simulink model "massbalancer3"  (R2024a)
settings: Solver=ode45  StartTime=0.0  StopTime=300  MaxStep=0.5  RelTol=1e-3
libraries: matrix_library x29, sharedutil x3, sharedtransform x2, dspinverses x1, aerolibutil x1
(part 2 of 3)

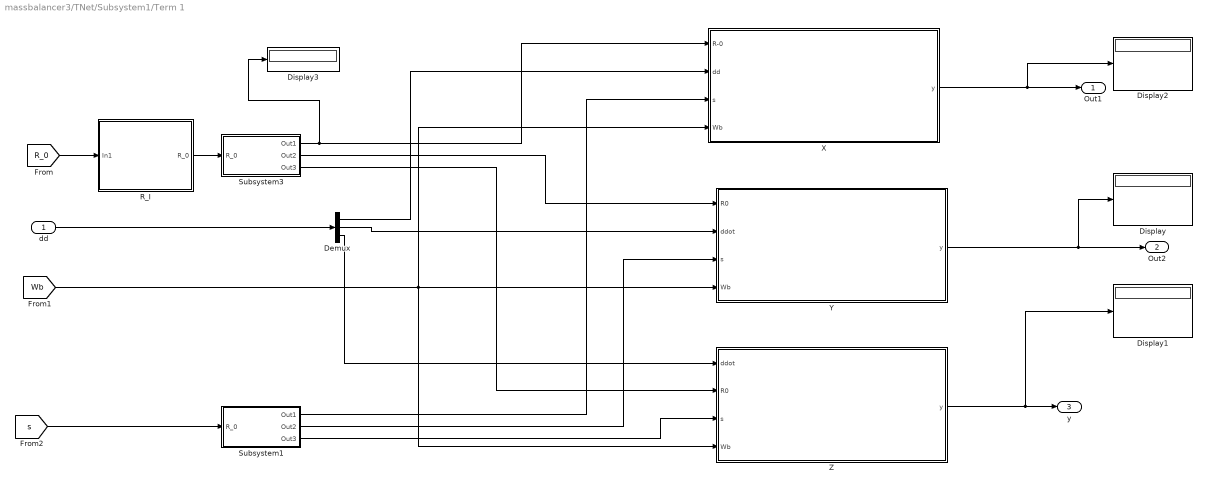
== system massbalancer3/TNet/Subsystem1/Term 1 ==
  dd : Inport
  Demux : Demux  Outputs=3
  Display{,1..3} (4 alike) : Display
  R_I : Subsystem
  Subsystem1 : Subsystem
  Subsystem3 : Subsystem
  X : Subsystem
  Y : Subsystem
  Z : Subsystem
  Out1 : Outport
  Out2 : Outport  Port=2
  y : Outport  Port=3
  wires:
  [R_0] -> R_I/1(In1)
  [s] -> Subsystem1/1(R_0)
  Demux/1 -> X/2(dd)
  R_I/1(R_0) -> Subsystem3/1(R_0)
  Subsystem3/1(Out1) -> X/1(R-0), Display3/1
  Subsystem1/2(Out2) -> Y/3(s)
  Subsystem1/1(Out1) -> X/3(s)
  Subsystem1/3(Out3) -> Z/3(s)
  Subsystem3/3(Out3) -> Z/2(R0)
  dd/1 -> Demux/1
  Subsystem3/2(Out2) -> Y/1(R0)
  Demux/3 -> Z/1(ddot)
  [Wb] -> X/4(Wb), Z/4(Wb), Y/4(Wb)
  Y/1(y) -> Display/1, Out2/1
  X/1(y) -> Display2/1, Out1/1
  Demux/2 -> Y/2(ddot)
  Z/1(y) -> Display1/1, y/1

== system massbalancer3/TNet/Subsystem1/Term2 ==
  dd : Inport
  Demux : Demux  Outputs=3
  Display : Display
  R_I : Subsystem
  Subsystem1 : Subsystem
  Subsystem3 : Subsystem
  X : Subsystem
  Y : Subsystem
  Z : Subsystem
  Output : Outport
  Output1 : Outport  Port=2
  Output2 : Outport  Port=3
  wires:
  Subsystem1/1(Out1) -> X/3(s)
  Demux/1 -> X/2(Ddot)
  dd/1 -> Demux/1
  Subsystem3/1(Out1) -> X/1(R-0)
  Demux/2 -> Y/2(ddot)
  Subsystem3/3(Out3) -> Z/2(R0)
  Subsystem3/2(Out2) -> Y/1(R0)
  [Wb] -> Z/4(Wb), X/4(Wb), Y/4(Wb)
  Demux/3 -> Z/1(ddot)
  [s] -> Subsystem1/1(R_0)
  Subsystem1/2(Out2) -> Y/3(s)
  [R_0] -> R_I/1(In1)
  Subsystem1/3(Out3) -> Z/3(s)
  X/1(Output) -> Output/1
  Y/1(Output) -> Display/1, Output1/1
  Z/1(Output1) -> Output2/1
  R_I/1(R_0) -> Subsystem3/1(R_0)

== system massbalancer3/TNet/Subsystem1/Term3 ==
  Input : Inport
  Demux : Demux  Outputs=3
  Display{,1..3} (4 alike) : Display
  Subsystem1 : Subsystem
  Subsystem3 : Subsystem
  X : Subsystem
  Y : Subsystem
  Z : Subsystem
  Output : Outport
  Output1 : Outport  Port=2
  Output2 : Outport  Port=3
  wires:
  Subsystem3/1(Out1) -> X/3(r)
  Subsystem3/2(Out2) -> Y/3(r)
  Subsystem3/3(Out3) -> Z/1(r)
  Demux/1 -> X/1(ddoubledot)
  Demux/2 -> Y/1(ddoubledot)
  Demux/3 -> Z/3(ddoubledot)
  [s] -> Subsystem1/1(R_0)
  Subsystem1/1(Out1) -> X/2(s)
  Subsystem1/2(Out2) -> Y/2(s)
  Subsystem1/3(Out3) -> Z/2(s)
  X/1(y) -> Display2/1, Output/1
  Y/1(y) -> Display/1, Output1/1
  Z/1(y) -> Display1/1, Output2/1
  [R_0] -> Subsystem3/1(R_0), Display3/1
  Input/1 -> Demux/1

== system massbalancer3/TNet/TBalances/R_I ==
  In1 : Inport
  Add : Sum
  Matrix Concatenate1 : Concatenate  NumInputs=3  Mode=Multidimensional array  ConcatenateDimension=2
  Product : Product
  Product1 : Product
  Product2 : Product
  Selector : Selector  InputPortWidth=3  IndexOptions=Index vector (dialog)  Indices=[1]  OutputSizes=1
  Selector1 : Selector  InputPortWidth=3  IndexOptions=Index vector (dialog)  Indices=[2]  OutputSizes=1
  Selector2 : Selector  InputPortWidth=3  IndexOptions=Index vector (dialog)  Indices=[3]  OutputSizes=1
  Subsystem3 : Subsystem
  Subsystem4 : Subsystem
  Sum1 : Sum  Inputs=|++
  Sum2 : Sum  Inputs=|++
  R_0 : Outport
  wires:
  Subsystem4/1(Out1) -> Add/1
  Product1/1 -> Sum1/1
  Selector1/1 -> Product1/1
  Selector/1 -> Product/1
  Subsystem3/2(Out2) -> Product1/2
  Selector2/1 -> Product2/1
  Subsystem4/2(Out2) -> Sum1/2
  In1/1 -> Selector/1, Selector1/1, Selector2/1
  Subsystem4/3(Out3) -> Sum2/2
  Product/1 -> Add/2
  Subsystem3/1(Out1) -> Product/2
  [S] -> Subsystem3/1(In1)
  Subsystem3/3(Out3) -> Product2/2
  Product2/1 -> Sum2/1
  [R_0] -> Subsystem4/1(In1)
  Add/1 -> Matrix Concatenate1/1
  Sum1/1 -> Matrix Concatenate1/2
  Sum2/1 -> Matrix Concatenate1/3
  Matrix Concatenate1/1 -> R_0/1

== system massbalancer3/TNet/TBalances/Term1 ==
  dd : Inport
  S : Inport  Port=2
  R_0 : Inport  Port=3
  Wb : Inport  Port=4
  Demux : Demux  Outputs=3
  Subsystem1 : Subsystem
  Subsystem3 : Subsystem
  X : Subsystem
  Y : Subsystem
  Z : Subsystem
  Output : Outport
  Output1 : Outport  Port=2
  Output2 : Outport  Port=3
  wires:
  R_0/1 -> Subsystem3/1(R_0)
  Subsystem3/1(Out1) -> X/1(R-0)
  Subsystem3/2(Out2) -> Y/1(R0)
  Subsystem3/3(Out3) -> Z/2(R0)
  dd/1 -> Demux/1
  Demux/1 -> X/2(dd)
  Demux/2 -> Y/2(ddot)
  Wb/1 -> Z/4(Wb), X/4(Wb), Y/4(Wb)
  Demux/3 -> Z/1(ddot)
  S/1 -> Subsystem1/1(R_0)
  Subsystem1/1(Out1) -> X/3(s)
  Subsystem1/2(Out2) -> Y/3(s)
  Subsystem1/3(Out3) -> Z/3(s)
  X/1(y) -> Output/1
  Y/1(y) -> Output1/1
  Z/1(y) -> Output2/1

== system massbalancer3/TNet/TBalances/Term2 ==
  ddot : Inport
  r0 : Inport  Port=2
  s : Inport  Port=3
  wb : Inport  Port=4
  Demux : Demux  Outputs=3
  Display : Display
  Display2 : Display
  Subsystem1 : Subsystem
  Subsystem3 : Subsystem
  X : Subsystem
  Y : Subsystem
  Z : Subsystem
  Output : Outport
  Output1 : Outport  Port=2
  Output2 : Outport  Port=3
  wires:
  Subsystem1/1(Out1) -> X/3(s)
  Demux/1 -> X/2(Ddot)
  ddot/1 -> Demux/1
  Subsystem3/1(Out1) -> X/1(R-0)
  Demux/2 -> Y/2(ddot)
  Subsystem3/3(Out3) -> Z/2(R0)
  Subsystem3/2(Out2) -> Y/1(R0)
  wb/1 -> Z/4(Wb), X/4(Wb), Y/4(Wb)
  Demux/3 -> Z/1(ddot)
  s/1 -> Subsystem1/1(R_0)
  Subsystem1/2(Out2) -> Y/3(s)
  r0/1 -> Subsystem3/1(R_0)
  Subsystem1/3(Out3) -> Z/3(s)
  X/1(Output) -> Display2/1, Output/1
  Y/1(Output) -> Output1/1
  Z/1(Output1) -> Display/1, Output2/1

== system massbalancer3/TNet/TBalances/Term3 ==
  r : Inport
  ddoubledot : Inport  Port=2
  s : Inport  Port=3
  Demux : Demux  Outputs=3
  Display : Display
  Display1 : Display
  Display2 : Display
  Subsystem1 : Subsystem
  Subsystem3 : Subsystem
  X : Subsystem
  Y : Subsystem
  Z : Subsystem
  Output : Outport
  Output1 : Outport  Port=2
  Output2 : Outport  Port=3
  wires:
  r/1 -> Subsystem3/1(R_0)
  ddoubledot/1 -> Demux/1
  Subsystem3/1(Out1) -> X/3(r)
  Subsystem3/2(Out2) -> Y/3(r)
  Subsystem3/3(Out3) -> Z/1(r)
  Demux/1 -> X/1(ddoubledot)
  Demux/2 -> Y/1(ddoubledot)
  Demux/3 -> Z/3(ddoubledot)
  s/1 -> Subsystem1/1(R_0)
  Subsystem1/1(Out1) -> X/2(s)
  Subsystem1/2(Out2) -> Y/2(s)
  Subsystem1/3(Out3) -> Z/2(s)
  X/1(y) -> Display2/1, Output/1
  Y/1(y) -> Display/1, Output1/1
  Z/1(y) -> Display1/1, Output2/1

== system massbalancer3/TNet/Tbalances Init T Gravity /Fgravity ==
  Matrix Multiply : Product  Multiplication=Matrix(*)
  Q(q) rotational form of quaternio : Subsystem
  Out1 : Outport
  wires:
  Q(q) rotational form of quaternio/1(Out1) -> Matrix Multiply/1
  [G] -> Matrix Multiply/2
  [q] -> Q(q) rotational form of quaternio/1(Q_input)
  Matrix Multiply/1 -> Out1/1

== system massbalancer3/TNet/Tbalances Init T Gravity /Subsystem ==
  Subsystem2 : Subsystem
  Output : Outport
  wires:
  [M_r] -> Subsystem2/1(In1)
  Subsystem2/1(Output) -> Output/1

== system massbalancer3/Wdot b/I_r/Subsystem ==
  In1 : Inport
  Constant : Constant  Value=0  VectorParams1D=off
  Constant1 : Constant  Value=0  VectorParams1D=off
  Constant2 : Constant  Value=0  VectorParams1D=off
  Demux : Demux  Outputs=3
  Gain : Gain  Gain=-1
  Gain1 : Gain  Gain=-1
  Gain2 : Gain  Gain=-1
  Matrix Concatenate : Concatenate  NumInputs=3  Mode=Multidimensional array  ConcatenateDimension=2
  Mux : Mux  Inputs=3
  Mux1 : Mux  Inputs=3
  Mux2 : Mux  Inputs=3
  Out1 : Outport
  wires:
  Constant/1 -> Mux/1
  Gain2/1 -> Mux2/1
  Gain1/1 -> Mux1/3
  Mux/1 -> Matrix Concatenate/1
  Demux/2 -> Mux/3, Gain2/1
  In1/1 -> Demux/1
  Gain/1 -> Mux/2
  Demux/3 -> Mux1/1, Gain/1
  Mux1/1 -> Matrix Concatenate/2
  Mux2/1 -> Matrix Concatenate/3
  Demux/1 -> Mux2/2, Gain1/1
  Constant1/1 -> Mux1/2
  Constant2/1 -> Mux2/3
  Matrix Concatenate/1 -> Out1/1

== system massbalancer3/Wdot b/I_r/Subsystem1 ==
  In1 : Inport
  Constant : Constant  Value=0  VectorParams1D=off
  Constant1 : Constant  Value=0  VectorParams1D=off
  Constant2 : Constant  Value=0  VectorParams1D=off
  Demux : Demux  Outputs=3
  Gain : Gain  Gain=-1
  Gain1 : Gain  Gain=-1
  Gain2 : Gain  Gain=-1
  Matrix Concatenate : Concatenate  NumInputs=3  Mode=Multidimensional array  ConcatenateDimension=2
  Mux : Mux  Inputs=3
  Mux1 : Mux  Inputs=3
  Mux2 : Mux  Inputs=3
  Out1 : Outport
  wires:
  Matrix Concatenate/1 -> Out1/1
  Constant2/1 -> Mux2/3
  Constant1/1 -> Mux1/2
  Demux/1 -> Gain1/1, Mux2/2
  Mux2/1 -> Matrix Concatenate/3
  Mux1/1 -> Matrix Concatenate/2
  Demux/3 -> Gain/1, Mux1/1
  Gain/1 -> Mux/2
  In1/1 -> Demux/1
  Demux/2 -> Gain2/1, Mux/3
  Mux/1 -> Matrix Concatenate/1
  Gain1/1 -> Mux1/3
  Gain2/1 -> Mux2/1
  Constant/1 -> Mux/1

== system massbalancer3/Wdot b/I_r/Subsystem2 ==
  In1 : Inport
  Constant : Constant  Value=0  VectorParams1D=off
  Constant1 : Constant  Value=0  VectorParams1D=off
  Constant2 : Constant  Value=0  VectorParams1D=off
  Demux : Demux  Outputs=3
  Gain : Gain  Gain=-1
  Gain1 : Gain  Gain=-1
  Gain2 : Gain  Gain=-1
  Matrix Concatenate : Concatenate  NumInputs=3  Mode=Multidimensional array  ConcatenateDimension=2
  Mux : Mux  Inputs=3
  Mux1 : Mux  Inputs=3
  Mux2 : Mux  Inputs=3
  Out1 : Outport
  wires:
  Constant/1 -> Mux/1
  Gain2/1 -> Mux2/1
  Gain1/1 -> Mux1/3
  Mux/1 -> Matrix Concatenate/1
  Demux/2 -> Mux/3, Gain2/1
  In1/1 -> Demux/1
  Gain/1 -> Mux/2
  Demux/3 -> Mux1/1, Gain/1
  Mux1/1 -> Matrix Concatenate/2
  Mux2/1 -> Matrix Concatenate/3
  Demux/1 -> Mux2/2, Gain1/1
  Constant1/1 -> Mux1/2
  Constant2/1 -> Mux2/3
  Matrix Concatenate/1 -> Out1/1

== system massbalancer3/Wdot b/I_r/Subsystem3 ==
  In1 : Inport
  Reshape : Reshape  OutputDimensionality=Column vector (2-D)  OutputDimensions=[1,3]
  Selector : Selector  InputPortWidth=9  IndexOptions=Index vector (dialog)  Indices=[1]  OutputSizes=1
  Selector1 : Selector  InputPortWidth=9  IndexOptions=Index vector (dialog)  Indices=[2]  OutputSizes=1
  Selector2 : Selector  InputPortWidth=9  IndexOptions=Index vector (dialog)  Indices=[3]  OutputSizes=1
  Selector3 : Selector  InputPortWidth=9  IndexOptions=Index vector (dialog)  Indices=[4]  OutputSizes=1
  Selector4 : Selector  InputPortWidth=9  IndexOptions=Index vector (dialog)  Indices=[5]  OutputSizes=1
  Selector5 : Selector  InputPortWidth=9  IndexOptions=Index vector (dialog)  Indices=[6]  OutputSizes=1
  Selector6 : Selector  InputPortWidth=9  IndexOptions=Index vector (dialog)  Indices=[7]  OutputSizes=1
  Selector7 : Selector  InputPortWidth=9  IndexOptions=Index vector (dialog)  Indices=[8]  OutputSizes=1
  Selector8 : Selector  InputPortWidth=9  IndexOptions=Index vector (dialog)  Indices=[9]  OutputSizes=1
  Vector Concatenate : Concatenate  NumInputs=3  Mode=Multidimensional array
  Vector Concatenate1 : Concatenate  NumInputs=3  Mode=Multidimensional array
  Vector Concatenate2 : Concatenate  NumInputs=3  Mode=Multidimensional array
  Out1 : Outport
  Out2 : Outport  Port=2
  Out3 : Outport  Port=3
  wires:
  Selector2/1 -> Vector Concatenate/3
  Vector Concatenate/1 -> Out1/1
  Selector8/1 -> Vector Concatenate2/3
  Selector4/1 -> Vector Concatenate1/2
  Selector6/1 -> Vector Concatenate2/1
  In1/1 -> Reshape/1
  Reshape/1 -> Selector8/1, Selector7/1, Selector6/1, Selector5/1, Selector4/1, Selector3/1, Selector2/1, Selector1/1, Selector/1
  Selector/1 -> Vector Concatenate/1
  Selector5/1 -> Vector Concatenate1/3
  Selector7/1 -> Vector Concatenate2/2
  Vector Concatenate2/1 -> Out3/1
  Vector Concatenate1/1 -> Out2/1
  Selector1/1 -> Vector Concatenate/2
  Selector3/1 -> Vector Concatenate1/1

== system massbalancer3/Wdot b/I_r/Subsystem4 ==
  In1 : Inport
  Reshape : Reshape  OutputDimensionality=Column vector (2-D)  OutputDimensions=[1,3]
  Selector : Selector  InputPortWidth=9  IndexOptions=Index vector (dialog)  Indices=[1]  OutputSizes=1
  Selector1 : Selector  InputPortWidth=9  IndexOptions=Index vector (dialog)  Indices=[2]  OutputSizes=1
  Selector2 : Selector  InputPortWidth=9  IndexOptions=Index vector (dialog)  Indices=[3]  OutputSizes=1
  Selector3 : Selector  InputPortWidth=9  IndexOptions=Index vector (dialog)  Indices=[4]  OutputSizes=1
  Selector4 : Selector  InputPortWidth=9  IndexOptions=Index vector (dialog)  Indices=[5]  OutputSizes=1
  Selector5 : Selector  InputPortWidth=9  IndexOptions=Index vector (dialog)  Indices=[6]  OutputSizes=1
  Selector6 : Selector  InputPortWidth=9  IndexOptions=Index vector (dialog)  Indices=[7]  OutputSizes=1
  Selector7 : Selector  InputPortWidth=9  IndexOptions=Index vector (dialog)  Indices=[8]  OutputSizes=1
  Selector8 : Selector  InputPortWidth=9  IndexOptions=Index vector (dialog)  Indices=[9]  OutputSizes=1
  Vector Concatenate : Concatenate  NumInputs=3  Mode=Multidimensional array
  Vector Concatenate1 : Concatenate  NumInputs=3  Mode=Multidimensional array
  Vector Concatenate2 : Concatenate  NumInputs=3  Mode=Multidimensional array
  Out1 : Outport
  Out2 : Outport  Port=2
  Out3 : Outport  Port=3
  wires:
  Selector3/1 -> Vector Concatenate1/1
  Selector1/1 -> Vector Concatenate/2
  Vector Concatenate1/1 -> Out2/1
  Vector Concatenate2/1 -> Out3/1
  Selector7/1 -> Vector Concatenate2/2
  Selector5/1 -> Vector Concatenate1/3
  Selector/1 -> Vector Concatenate/1
  Reshape/1 -> Selector/1, Selector1/1, Selector2/1, Selector3/1, Selector4/1, Selector5/1, Selector6/1, Selector7/1, Selector8/1
  In1/1 -> Reshape/1
  Selector6/1 -> Vector Concatenate2/1
  Selector4/1 -> Vector Concatenate1/2
  Selector8/1 -> Vector Concatenate2/3
  Vector Concatenate/1 -> Out1/1
  Selector2/1 -> Vector Concatenate/3

== system massbalancer3/Subsystem1/Subsystem1/Subsystem/Enabled Subsystem ==
  In1 : Inport
  Enable : EnablePort
  Out1 : Outport
  wires:
  In1/1 -> Out1/1

== system massbalancer3/Subsystem1/Subsystem1/Subsystem1/Enabled Subsystem ==
  In1 : Inport
  Enable : EnablePort
  Out1 : Outport
  wires:
  In1/1 -> Out1/1

== system massbalancer3/Subsystem1/Subsystem2/Subsystem/Enabled Subsystem ==
  In1 : Inport
  Enable : EnablePort
  Out1 : Outport
  wires:
  In1/1 -> Out1/1

== system massbalancer3/Subsystem1/Subsystem2/Subsystem1/Enabled Subsystem ==
  In1 : Inport
  Enable : EnablePort
  Out1 : Outport
  wires:
  In1/1 -> Out1/1

== system massbalancer3/Subsystem1/Subsystem3/Subsystem/Enabled Subsystem ==
  In1 : Inport
  Enable : EnablePort
  Out1 : Outport
  wires:
  In1/1 -> Out1/1

== system massbalancer3/Subsystem1/Subsystem3/Subsystem1/Enabled Subsystem ==
  In1 : Inport
  Enable : EnablePort
  Out1 : Outport
  wires:
  In1/1 -> Out1/1

== system massbalancer3/Subsystem2/Subsystem1/Subsystem/Enabled Subsystem ==
  In1 : Inport
  Enable : EnablePort
  Out1 : Outport
  wires:
  In1/1 -> Out1/1

== system massbalancer3/Subsystem2/Subsystem2/Subsystem/Enabled Subsystem ==
  In1 : Inport
  Enable : EnablePort
  Out1 : Outport
  wires:
  In1/1 -> Out1/1

== system massbalancer3/Subsystem2/Subsystem3/Subsystem/Enabled Subsystem ==
  In1 : Inport
  Enable : EnablePort
  Out1 : Outport
  wires:
  In1/1 -> Out1/1

== system massbalancer3/TNet/Subsystem1/R_I/Subsystem3 ==
  In1 : Inport
  Reshape : Reshape  OutputDimensionality=Column vector (2-D)  OutputDimensions=[1,3]
  Selector : Selector  InputPortWidth=9  IndexOptions=Index vector (dialog)  Indices=[1]  OutputSizes=1
  Selector1 : Selector  InputPortWidth=9  IndexOptions=Index vector (dialog)  Indices=[2]  OutputSizes=1
  Selector2 : Selector  InputPortWidth=9  IndexOptions=Index vector (dialog)  Indices=[3]  OutputSizes=1
  Selector3 : Selector  InputPortWidth=9  IndexOptions=Index vector (dialog)  Indices=[4]  OutputSizes=1
  Selector4 : Selector  InputPortWidth=9  IndexOptions=Index vector (dialog)  Indices=[5]  OutputSizes=1
  Selector5 : Selector  InputPortWidth=9  IndexOptions=Index vector (dialog)  Indices=[6]  OutputSizes=1
  Selector6 : Selector  InputPortWidth=9  IndexOptions=Index vector (dialog)  Indices=[7]  OutputSizes=1
  Selector7 : Selector  InputPortWidth=9  IndexOptions=Index vector (dialog)  Indices=[8]  OutputSizes=1
  Selector8 : Selector  InputPortWidth=9  IndexOptions=Index vector (dialog)  Indices=[9]  OutputSizes=1
  Vector Concatenate : Concatenate  NumInputs=3  Mode=Multidimensional array
  Vector Concatenate1 : Concatenate  NumInputs=3  Mode=Multidimensional array
  Vector Concatenate2 : Concatenate  NumInputs=3  Mode=Multidimensional array
  Out1 : Outport
  Out2 : Outport  Port=2
  Out3 : Outport  Port=3
  wires:
  Selector2/1 -> Vector Concatenate/3
  Vector Concatenate/1 -> Out1/1
  Selector8/1 -> Vector Concatenate2/3
  Selector4/1 -> Vector Concatenate1/2
  Selector6/1 -> Vector Concatenate2/1
  In1/1 -> Reshape/1
  Reshape/1 -> Selector8/1, Selector7/1, Selector6/1, Selector5/1, Selector4/1, Selector3/1, Selector2/1, Selector1/1, Selector/1
  Selector/1 -> Vector Concatenate/1
  Selector5/1 -> Vector Concatenate1/3
  Selector7/1 -> Vector Concatenate2/2
  Vector Concatenate2/1 -> Out3/1
  Vector Concatenate1/1 -> Out2/1
  Selector1/1 -> Vector Concatenate/2
  Selector3/1 -> Vector Concatenate1/1

== system massbalancer3/TNet/Subsystem1/R_I/Subsystem4 ==
  In1 : Inport
  Reshape : Reshape  OutputDimensionality=Column vector (2-D)  OutputDimensions=[1,3]
  Selector : Selector  InputPortWidth=9  IndexOptions=Index vector (dialog)  Indices=[1]  OutputSizes=1
  Selector1 : Selector  InputPortWidth=9  IndexOptions=Index vector (dialog)  Indices=[2]  OutputSizes=1
  Selector2 : Selector  InputPortWidth=9  IndexOptions=Index vector (dialog)  Indices=[3]  OutputSizes=1
  Selector3 : Selector  InputPortWidth=9  IndexOptions=Index vector (dialog)  Indices=[4]  OutputSizes=1
  Selector4 : Selector  InputPortWidth=9  IndexOptions=Index vector (dialog)  Indices=[5]  OutputSizes=1
  Selector5 : Selector  InputPortWidth=9  IndexOptions=Index vector (dialog)  Indices=[6]  OutputSizes=1
  Selector6 : Selector  InputPortWidth=9  IndexOptions=Index vector (dialog)  Indices=[7]  OutputSizes=1
  Selector7 : Selector  InputPortWidth=9  IndexOptions=Index vector (dialog)  Indices=[8]  OutputSizes=1
  Selector8 : Selector  InputPortWidth=9  IndexOptions=Index vector (dialog)  Indices=[9]  OutputSizes=1
  Vector Concatenate : Concatenate  NumInputs=3  Mode=Multidimensional array
  Vector Concatenate1 : Concatenate  NumInputs=3  Mode=Multidimensional array
  Vector Concatenate2 : Concatenate  NumInputs=3  Mode=Multidimensional array
  Out1 : Outport
  Out2 : Outport  Port=2
  Out3 : Outport  Port=3
  wires:
  Selector3/1 -> Vector Concatenate1/1
  Selector1/1 -> Vector Concatenate/2
  Vector Concatenate1/1 -> Out2/1
  Vector Concatenate2/1 -> Out3/1
  Selector7/1 -> Vector Concatenate2/2
  Selector5/1 -> Vector Concatenate1/3
  Selector/1 -> Vector Concatenate/1
  Reshape/1 -> Selector/1, Selector1/1, Selector2/1, Selector3/1, Selector4/1, Selector5/1, Selector6/1, Selector7/1, Selector8/1
  In1/1 -> Reshape/1
  Selector6/1 -> Vector Concatenate2/1
  Selector4/1 -> Vector Concatenate1/2
  Selector8/1 -> Vector Concatenate2/3
  Vector Concatenate/1 -> Out1/1
  Selector2/1 -> Vector Concatenate/3

== system massbalancer3/TNet/Subsystem1/Tbalances Init T Gravity /Fgravity ==
  Display : Display
  Matrix Multiply : Product  Multiplication=Matrix(*)
  Q(q) rotational form of quaternio : Subsystem
  Out1 : Outport
  wires:
  Q(q) rotational form of quaternio/1(Out1) -> Matrix Multiply/1
  [G] -> Matrix Multiply/2
  [q] -> Q(q) rotational form of quaternio/1(Q_input)
  Matrix Multiply/1 -> Display/1, Out1/1

== system massbalancer3/TNet/Subsystem1/Tbalances Init T Gravity /Subsystem ==
  Output : Outport
  wires:
  [M_r] -> Output/1

== system massbalancer3/TNet/Subsystem1/Tbalances Init T Gravity /Subsystem1 ==
  In1 : Inport
  Constant : Constant  Value=0  VectorParams1D=off
  Constant1 : Constant  Value=0  VectorParams1D=off
  Constant2 : Constant  Value=0  VectorParams1D=off
  Demux : Demux  Outputs=3
  Gain : Gain  Gain=-1
  Gain1 : Gain  Gain=-1
  Gain2 : Gain  Gain=-1
  Matrix Concatenate : Concatenate  NumInputs=3  Mode=Multidimensional array  ConcatenateDimension=2
  Mux : Mux  Inputs=3
  Mux1 : Mux  Inputs=3
  Mux2 : Mux  Inputs=3
  Out1 : Outport
  wires:
  Constant/1 -> Mux/1
  Gain2/1 -> Mux2/1
  Gain1/1 -> Mux1/3
  Mux/1 -> Matrix Concatenate/1
  Demux/2 -> Mux/3, Gain2/1
  In1/1 -> Demux/1
  Gain/1 -> Mux/2
  Demux/3 -> Mux1/1, Gain/1
  Mux1/1 -> Matrix Concatenate/2
  Mux2/1 -> Matrix Concatenate/3
  Demux/1 -> Mux2/2, Gain1/1
  Constant1/1 -> Mux1/2
  Constant2/1 -> Mux2/3
  Matrix Concatenate/1 -> Out1/1

== system massbalancer3/TNet/Subsystem1/Term 1/R_I ==
  In1 : Inport
  Add : Sum
  Displacment D : Constant  Value=[0.05;-0.03;0.02]  VectorParams1D=off
  Matrix Concatenate1 : Concatenate  NumInputs=3  Mode=Multidimensional array  ConcatenateDimension=2
  Product : Product
  Product1 : Product
  Product2 : Product
  S value : Constant  Value=|
      | [ 0.9535,  0.2760,  0.0953;
      |       0.0953,  0.9206,  0.2859;
      |       0.2859,  0.2760,  0.9535 ]
  Selector : Selector  InputPortWidth=3  IndexOptions=Index vector (dialog)  Indices=[1]  OutputSizes=1
  Selector1 : Selector  InputPortWidth=3  IndexOptions=Index vector (dialog)  Indices=[2]  OutputSizes=1
  Selector2 : Selector  InputPortWidth=3  IndexOptions=Index vector (dialog)  Indices=[3]  OutputSizes=1
  Subsystem3 : Subsystem
  Subsystem4 : Subsystem
  Sum1 : Sum  Inputs=|++
  Sum2 : Sum  Inputs=|++
  R_0 : Outport
  wires:
  Subsystem4/1(Out1) -> Add/1
  Product1/1 -> Sum1/1
  Selector1/1 -> Product1/1
  Selector/1 -> Product/1
  Subsystem3/2(Out2) -> Product1/2
  Selector2/1 -> Product2/1
  Subsystem4/2(Out2) -> Sum1/2
  Displacment D/1 -> Selector/1, Selector1/1, Selector2/1
  Subsystem4/3(Out3) -> Sum2/2
  Product/1 -> Add/2
  Subsystem3/1(Out1) -> Product/2
  S value/1 -> Subsystem3/1(In1)
  Subsystem3/3(Out3) -> Product2/2
  Product2/1 -> Sum2/1
  In1/1 -> Subsystem4/1(In1)
  Add/1 -> Matrix Concatenate1/1
  Sum1/1 -> Matrix Concatenate1/2
  Sum2/1 -> Matrix Concatenate1/3
  Matrix Concatenate1/1 -> R_0/1

== system massbalancer3/TNet/Subsystem1/Term 1/Subsystem1 ==
  R_0 : Inport
  Reshape : Reshape  OutputDimensionality=Column vector (2-D)  OutputDimensions=[1,3]
  Selector : Selector  InputPortWidth=9  IndexOptions=Index vector (dialog)  Indices=[1]  OutputSizes=1
  Selector1 : Selector  InputPortWidth=9  IndexOptions=Index vector (dialog)  Indices=[2]  OutputSizes=1
  Selector2 : Selector  InputPortWidth=9  IndexOptions=Index vector (dialog)  Indices=[3]  OutputSizes=1
  Selector3 : Selector  InputPortWidth=9  IndexOptions=Index vector (dialog)  Indices=[4]  OutputSizes=1
  Selector4 : Selector  InputPortWidth=9  IndexOptions=Index vector (dialog)  Indices=[5]  OutputSizes=1
  Selector5 : Selector  InputPortWidth=9  IndexOptions=Index vector (dialog)  Indices=[6]  OutputSizes=1
  Selector6 : Selector  InputPortWidth=9  IndexOptions=Index vector (dialog)  Indices=[7]  OutputSizes=1
  Selector7 : Selector  InputPortWidth=9  IndexOptions=Index vector (dialog)  Indices=[8]  OutputSizes=1
  Selector8 : Selector  InputPortWidth=9  IndexOptions=Index vector (dialog)  Indices=[9]  OutputSizes=1
  Vector Concatenate : Concatenate  NumInputs=3  Mode=Multidimensional array
  Vector Concatenate1 : Concatenate  NumInputs=3  Mode=Multidimensional array
  Vector Concatenate2 : Concatenate  NumInputs=3  Mode=Multidimensional array
  Out1 : Outport
  Out2 : Outport  Port=2
  Out3 : Outport  Port=3
  wires:
  Selector3/1 -> Vector Concatenate1/1
  Selector1/1 -> Vector Concatenate/2
  Vector Concatenate1/1 -> Out2/1
  Vector Concatenate2/1 -> Out3/1
  Selector7/1 -> Vector Concatenate2/2
  Selector5/1 -> Vector Concatenate1/3
  Selector/1 -> Vector Concatenate/1
  Reshape/1 -> Selector/1, Selector1/1, Selector2/1, Selector3/1, Selector4/1, Selector5/1, Selector6/1, Selector7/1, Selector8/1
  R_0/1 -> Reshape/1
  Selector6/1 -> Vector Concatenate2/1
  Selector4/1 -> Vector Concatenate1/2
  Selector8/1 -> Vector Concatenate2/3
  Vector Concatenate/1 -> Out1/1
  Selector2/1 -> Vector Concatenate/3

== system massbalancer3/TNet/Subsystem1/Term 1/Subsystem3 ==
  R_0 : Inport
  Reshape : Reshape  OutputDimensionality=Column vector (2-D)  OutputDimensions=[1,3]
  Selector : Selector  InputPortWidth=9  IndexOptions=Index vector (dialog)  Indices=[1]  OutputSizes=1
  Selector1 : Selector  InputPortWidth=9  IndexOptions=Index vector (dialog)  Indices=[2]  OutputSizes=1
  Selector2 : Selector  InputPortWidth=9  IndexOptions=Index vector (dialog)  Indices=[3]  OutputSizes=1
  Selector3 : Selector  InputPortWidth=9  IndexOptions=Index vector (dialog)  Indices=[4]  OutputSizes=1
  Selector4 : Selector  InputPortWidth=9  IndexOptions=Index vector (dialog)  Indices=[5]  OutputSizes=1
  Selector5 : Selector  InputPortWidth=9  IndexOptions=Index vector (dialog)  Indices=[6]  OutputSizes=1
  Selector6 : Selector  InputPortWidth=9  IndexOptions=Index vector (dialog)  Indices=[7]  OutputSizes=1
  Selector7 : Selector  InputPortWidth=9  IndexOptions=Index vector (dialog)  Indices=[8]  OutputSizes=1
  Selector8 : Selector  InputPortWidth=9  IndexOptions=Index vector (dialog)  Indices=[9]  OutputSizes=1
  Vector Concatenate : Concatenate  NumInputs=3  Mode=Multidimensional array
  Vector Concatenate1 : Concatenate  NumInputs=3  Mode=Multidimensional array
  Vector Concatenate2 : Concatenate  NumInputs=3  Mode=Multidimensional array
  Out1 : Outport
  Out2 : Outport  Port=2
  Out3 : Outport  Port=3
  wires:
  Selector2/1 -> Vector Concatenate/3
  Vector Concatenate/1 -> Out1/1
  Selector8/1 -> Vector Concatenate2/3
  Selector4/1 -> Vector Concatenate1/2
  Selector6/1 -> Vector Concatenate2/1
  R_0/1 -> Reshape/1
  Reshape/1 -> Selector8/1, Selector7/1, Selector6/1, Selector5/1, Selector4/1, Selector3/1, Selector2/1, Selector1/1, Selector/1
  Selector/1 -> Vector Concatenate/1
  Selector5/1 -> Vector Concatenate1/3
  Selector7/1 -> Vector Concatenate2/2
  Vector Concatenate2/1 -> Out3/1
  Vector Concatenate1/1 -> Out2/1
  Selector1/1 -> Vector Concatenate/2
  Selector3/1 -> Vector Concatenate1/1

== system massbalancer3/TNet/Subsystem1/Term 1/X ==
  R-0 : Inport
  dd : Inport  Port=2
  s : Inport  Port=3
  Wb : Inport  Port=4
  Matrix Multiply : Product  Multiplication=Matrix(*)
  Matrix Multiply1 : Product  Multiplication=Matrix(*)
  Product : Product
  Subsystem : Subsystem
  Subsystem1 : Subsystem
  y : Outport
  wires:
  s/1 -> Product/2
  dd/1 -> Product/1
  Product/1 -> Subsystem1/1(In1)
  R-0/1 -> Matrix Multiply/2
  Wb/1 -> Subsystem/1(Wb)
  Subsystem/1(Out1) -> Matrix Multiply/1
  Subsystem1/1(Out1) -> Matrix Multiply1/1
  Matrix Multiply1/1 -> y/1
  Matrix Multiply/1 -> Matrix Multiply1/2

== system massbalancer3/TNet/Subsystem1/Term 1/Y ==
  R0 : Inport
  ddot : Inport  Port=2
  s : Inport  Port=3
  Wb : Inport  Port=4
  Product : Product
  Product1 : Product  Multiplication=Matrix(*)
  Product2 : Product  Multiplication=Matrix(*)
  Subsystem : Subsystem
  Subsystem1 : Subsystem
  y : Outport
  wires:
  Wb/1 -> Subsystem1/1(In1)
  Product/1 -> Subsystem/1(In1)
  Product2/1 -> y/1
  ddot/1 -> Product/1
  s/1 -> Product/2
  R0/1 -> Product1/2
  Subsystem/1(Out1) -> Product2/1
  Subsystem1/1(Out1) -> Product1/1
  Product1/1 -> Product2/2

== system massbalancer3/TNet/Subsystem1/Term 1/Z ==
  ddot : Inport
  R0 : Inport  Port=2
  s : Inport  Port=3
  Wb : Inport  Port=4
  Product : Product
  Product1 : Product  Multiplication=Matrix(*)
  Product2 : Product  Multiplication=Matrix(*)
  Subsystem1 : Subsystem
  Subsystem2 : Subsystem
  y : Outport
  wires:
  Product2/1 -> y/1
  Product1/1 -> Product2/2
  ddot/1 -> Product/1
  s/1 -> Product/2
  Product/1 -> Subsystem1/1(In1)
  Wb/1 -> Subsystem2/1(In1)
  R0/1 -> Product1/2
  Subsystem1/1(Out1) -> Product2/1
  Subsystem2/1(Out1) -> Product1/1

== system massbalancer3/TNet/Subsystem1/Term2/R_I ==
  In1 : Inport
  Add : Sum
  Displacment D : Constant  Value=[0.05;-0.03;0.02]  VectorParams1D=off
  Matrix Concatenate1 : Concatenate  NumInputs=3  Mode=Multidimensional array  ConcatenateDimension=2
  Product : Product
  Product1 : Product
  Product2 : Product
  S value : Constant  Value=|
      | [ 0.9535,  0.2760,  0.0953;
      |       0.0953,  0.9206,  0.2859;
      |       0.2859,  0.2760,  0.9535 ]
  Selector : Selector  InputPortWidth=3  IndexOptions=Index vector (dialog)  Indices=[1]  OutputSizes=1
  Selector1 : Selector  InputPortWidth=3  IndexOptions=Index vector (dialog)  Indices=[2]  OutputSizes=1
  Selector2 : Selector  InputPortWidth=3  IndexOptions=Index vector (dialog)  Indices=[3]  OutputSizes=1
  Subsystem3 : Subsystem
  Subsystem4 : Subsystem
  Sum1 : Sum  Inputs=|++
  Sum2 : Sum  Inputs=|++
  R_0 : Outport
  wires:
  Subsystem4/1(Out1) -> Add/1
  Product1/1 -> Sum1/1
  Selector1/1 -> Product1/1
  Selector/1 -> Product/1
  Subsystem3/2(Out2) -> Product1/2
  Selector2/1 -> Product2/1
  Subsystem4/2(Out2) -> Sum1/2
  Displacment D/1 -> Selector/1, Selector1/1, Selector2/1
  Subsystem4/3(Out3) -> Sum2/2
  Product/1 -> Add/2
  Subsystem3/1(Out1) -> Product/2
  S value/1 -> Subsystem3/1(In1)
  Subsystem3/3(Out3) -> Product2/2
  Product2/1 -> Sum2/1
  In1/1 -> Subsystem4/1(In1)
  Add/1 -> Matrix Concatenate1/1
  Sum1/1 -> Matrix Concatenate1/2
  Sum2/1 -> Matrix Concatenate1/3
  Matrix Concatenate1/1 -> R_0/1

== system massbalancer3/TNet/Subsystem1/Term2/Subsystem1 ==
  R_0 : Inport
  Reshape : Reshape  OutputDimensionality=Column vector (2-D)  OutputDimensions=[1,3]
  Selector : Selector  InputPortWidth=9  IndexOptions=Index vector (dialog)  Indices=[1]  OutputSizes=1
  Selector1 : Selector  InputPortWidth=9  IndexOptions=Index vector (dialog)  Indices=[2]  OutputSizes=1
  Selector2 : Selector  InputPortWidth=9  IndexOptions=Index vector (dialog)  Indices=[3]  OutputSizes=1
  Selector3 : Selector  InputPortWidth=9  IndexOptions=Index vector (dialog)  Indices=[4]  OutputSizes=1
  Selector4 : Selector  InputPortWidth=9  IndexOptions=Index vector (dialog)  Indices=[5]  OutputSizes=1
  Selector5 : Selector  InputPortWidth=9  IndexOptions=Index vector (dialog)  Indices=[6]  OutputSizes=1
  Selector6 : Selector  InputPortWidth=9  IndexOptions=Index vector (dialog)  Indices=[7]  OutputSizes=1
  Selector7 : Selector  InputPortWidth=9  IndexOptions=Index vector (dialog)  Indices=[8]  OutputSizes=1
  Selector8 : Selector  InputPortWidth=9  IndexOptions=Index vector (dialog)  Indices=[9]  OutputSizes=1
  Vector Concatenate : Concatenate  NumInputs=3  Mode=Multidimensional array
  Vector Concatenate1 : Concatenate  NumInputs=3  Mode=Multidimensional array
  Vector Concatenate2 : Concatenate  NumInputs=3  Mode=Multidimensional array
  Out1 : Outport
  Out2 : Outport  Port=2
  Out3 : Outport  Port=3
  wires:
  Selector3/1 -> Vector Concatenate1/1
  Selector1/1 -> Vector Concatenate/2
  Vector Concatenate1/1 -> Out2/1
  Vector Concatenate2/1 -> Out3/1
  Selector7/1 -> Vector Concatenate2/2
  Selector5/1 -> Vector Concatenate1/3
  Selector/1 -> Vector Concatenate/1
  Reshape/1 -> Selector/1, Selector1/1, Selector2/1, Selector3/1, Selector4/1, Selector5/1, Selector6/1, Selector7/1, Selector8/1
  R_0/1 -> Reshape/1
  Selector6/1 -> Vector Concatenate2/1
  Selector4/1 -> Vector Concatenate1/2
  Selector8/1 -> Vector Concatenate2/3
  Vector Concatenate/1 -> Out1/1
  Selector2/1 -> Vector Concatenate/3

== system massbalancer3/TNet/Subsystem1/Term2/Subsystem3 ==
  R_0 : Inport
  Reshape : Reshape  OutputDimensionality=Column vector (2-D)  OutputDimensions=[1,3]
  Selector : Selector  InputPortWidth=9  IndexOptions=Index vector (dialog)  Indices=[1]  OutputSizes=1
  Selector1 : Selector  InputPortWidth=9  IndexOptions=Index vector (dialog)  Indices=[2]  OutputSizes=1
  Selector2 : Selector  InputPortWidth=9  IndexOptions=Index vector (dialog)  Indices=[3]  OutputSizes=1
  Selector3 : Selector  InputPortWidth=9  IndexOptions=Index vector (dialog)  Indices=[4]  OutputSizes=1
  Selector4 : Selector  InputPortWidth=9  IndexOptions=Index vector (dialog)  Indices=[5]  OutputSizes=1
  Selector5 : Selector  InputPortWidth=9  IndexOptions=Index vector (dialog)  Indices=[6]  OutputSizes=1
  Selector6 : Selector  InputPortWidth=9  IndexOptions=Index vector (dialog)  Indices=[7]  OutputSizes=1
  Selector7 : Selector  InputPortWidth=9  IndexOptions=Index vector (dialog)  Indices=[8]  OutputSizes=1
  Selector8 : Selector  InputPortWidth=9  IndexOptions=Index vector (dialog)  Indices=[9]  OutputSizes=1
  Vector Concatenate : Concatenate  NumInputs=3  Mode=Multidimensional array
  Vector Concatenate1 : Concatenate  NumInputs=3  Mode=Multidimensional array
  Vector Concatenate2 : Concatenate  NumInputs=3  Mode=Multidimensional array
  Out1 : Outport
  Out2 : Outport  Port=2
  Out3 : Outport  Port=3
  wires:
  Selector2/1 -> Vector Concatenate/3
  Vector Concatenate/1 -> Out1/1
  Selector8/1 -> Vector Concatenate2/3
  Selector4/1 -> Vector Concatenate1/2
  Selector6/1 -> Vector Concatenate2/1
  R_0/1 -> Reshape/1
  Reshape/1 -> Selector8/1, Selector7/1, Selector6/1, Selector5/1, Selector4/1, Selector3/1, Selector2/1, Selector1/1, Selector/1
  Selector/1 -> Vector Concatenate/1
  Selector5/1 -> Vector Concatenate1/3
  Selector7/1 -> Vector Concatenate2/2
  Vector Concatenate2/1 -> Out3/1
  Vector Concatenate1/1 -> Out2/1
  Selector1/1 -> Vector Concatenate/2
  Selector3/1 -> Vector Concatenate1/1

== system massbalancer3/TNet/Subsystem1/Term2/X ==
  R-0 : Inport
  Ddot : Inport  Port=2
  s : Inport  Port=3
  Wb : Inport  Port=4
  Cross Product : matrix_library/Cross Product
  Cross Product1 : matrix_library/Cross Product
  Display{,1..5} (6 alike) : Display
  Product : Product
  Output : Outport
  wires:
  Cross Product1/1 -> Display/1, Output/1
  R-0/1 -> Cross Product1/1
  Product/1 -> Cross Product/2, Display1/1
  s/1 -> Display4/1, Product/2
  Ddot/1 -> Display5/1, Product/1
  Wb/1 -> Cross Product/1, Display3/1
  Cross Product/1 -> Display2/1, Cross Product1/2

== system massbalancer3/TNet/Subsystem1/Term2/Y ==
  R0 : Inport
  ddot : Inport  Port=2
  s : Inport  Port=3
  Wb : Inport  Port=4
  Cross Product : matrix_library/Cross Product
  Cross Product1 : matrix_library/Cross Product
  Product : Product
  Output : Outport
  wires:
  s/1 -> Product/1
  Product/1 -> Cross Product/2
  R0/1 -> Cross Product1/1
  Cross Product/1 -> Cross Product1/2
  ddot/1 -> Product/2
  Wb/1 -> Cross Product/1
  Cross Product1/1 -> Output/1

== system massbalancer3/TNet/Subsystem1/Term2/Z ==
  ddot : Inport
  R0 : Inport  Port=2
  s : Inport  Port=3
  Wb : Inport  Port=4
  Cross Product : matrix_library/Cross Product
  Cross Product1 : matrix_library/Cross Product
  Product : Product
  Output1 : Outport
  wires:
  s/1 -> Product/1
  Product/1 -> Cross Product/2
  R0/1 -> Cross Product1/1
  Cross Product/1 -> Cross Product1/2
  ddot/1 -> Product/2
  Wb/1 -> Cross Product/1
  Cross Product1/1 -> Output1/1

== system massbalancer3/TNet/Subsystem1/Term3/Subsystem1 ==
  R_0 : Inport
  Reshape : Reshape  OutputDimensionality=Column vector (2-D)  OutputDimensions=[1,3]
  Selector : Selector  InputPortWidth=9  IndexOptions=Index vector (dialog)  Indices=[1]  OutputSizes=1
  Selector1 : Selector  InputPortWidth=9  IndexOptions=Index vector (dialog)  Indices=[2]  OutputSizes=1
  Selector2 : Selector  InputPortWidth=9  IndexOptions=Index vector (dialog)  Indices=[3]  OutputSizes=1
  Selector3 : Selector  InputPortWidth=9  IndexOptions=Index vector (dialog)  Indices=[4]  OutputSizes=1
  Selector4 : Selector  InputPortWidth=9  IndexOptions=Index vector (dialog)  Indices=[5]  OutputSizes=1
  Selector5 : Selector  InputPortWidth=9  IndexOptions=Index vector (dialog)  Indices=[6]  OutputSizes=1
  Selector6 : Selector  InputPortWidth=9  IndexOptions=Index vector (dialog)  Indices=[7]  OutputSizes=1
  Selector7 : Selector  InputPortWidth=9  IndexOptions=Index vector (dialog)  Indices=[8]  OutputSizes=1
  Selector8 : Selector  InputPortWidth=9  IndexOptions=Index vector (dialog)  Indices=[9]  OutputSizes=1
  Vector Concatenate : Concatenate  NumInputs=3  Mode=Multidimensional array
  Vector Concatenate1 : Concatenate  NumInputs=3  Mode=Multidimensional array
  Vector Concatenate2 : Concatenate  NumInputs=3  Mode=Multidimensional array
  Out1 : Outport
  Out2 : Outport  Port=2
  Out3 : Outport  Port=3
  wires:
  Selector3/1 -> Vector Concatenate1/1
  Selector1/1 -> Vector Concatenate/2
  Vector Concatenate1/1 -> Out2/1
  Vector Concatenate2/1 -> Out3/1
  Selector7/1 -> Vector Concatenate2/2
  Selector5/1 -> Vector Concatenate1/3
  Selector/1 -> Vector Concatenate/1
  Reshape/1 -> Selector/1, Selector1/1, Selector2/1, Selector3/1, Selector4/1, Selector5/1, Selector6/1, Selector7/1, Selector8/1
  R_0/1 -> Reshape/1
  Selector6/1 -> Vector Concatenate2/1
  Selector4/1 -> Vector Concatenate1/2
  Selector8/1 -> Vector Concatenate2/3
  Vector Concatenate/1 -> Out1/1
  Selector2/1 -> Vector Concatenate/3

== system massbalancer3/TNet/Subsystem1/Term3/Subsystem3 ==
  R_0 : Inport
  Reshape : Reshape  OutputDimensionality=Column vector (2-D)  OutputDimensions=[1,3]
  Selector : Selector  InputPortWidth=9  IndexOptions=Index vector (dialog)  Indices=[1]  OutputSizes=1
  Selector1 : Selector  InputPortWidth=9  IndexOptions=Index vector (dialog)  Indices=[2]  OutputSizes=1
  Selector2 : Selector  InputPortWidth=9  IndexOptions=Index vector (dialog)  Indices=[3]  OutputSizes=1
  Selector3 : Selector  InputPortWidth=9  IndexOptions=Index vector (dialog)  Indices=[4]  OutputSizes=1
  Selector4 : Selector  InputPortWidth=9  IndexOptions=Index vector (dialog)  Indices=[5]  OutputSizes=1
  Selector5 : Selector  InputPortWidth=9  IndexOptions=Index vector (dialog)  Indices=[6]  OutputSizes=1
  Selector6 : Selector  InputPortWidth=9  IndexOptions=Index vector (dialog)  Indices=[7]  OutputSizes=1
  Selector7 : Selector  InputPortWidth=9  IndexOptions=Index vector (dialog)  Indices=[8]  OutputSizes=1
  Selector8 : Selector  InputPortWidth=9  IndexOptions=Index vector (dialog)  Indices=[9]  OutputSizes=1
  Vector Concatenate : Concatenate  NumInputs=3  Mode=Multidimensional array
  Vector Concatenate1 : Concatenate  NumInputs=3  Mode=Multidimensional array
  Vector Concatenate2 : Concatenate  NumInputs=3  Mode=Multidimensional array
  Out1 : Outport
  Out2 : Outport  Port=2
  Out3 : Outport  Port=3
  wires:
  Selector2/1 -> Vector Concatenate/3
  Vector Concatenate/1 -> Out1/1
  Selector8/1 -> Vector Concatenate2/3
  Selector4/1 -> Vector Concatenate1/2
  Selector6/1 -> Vector Concatenate2/1
  R_0/1 -> Reshape/1
  Reshape/1 -> Selector8/1, Selector7/1, Selector6/1, Selector5/1, Selector4/1, Selector3/1, Selector2/1, Selector1/1, Selector/1
  Selector/1 -> Vector Concatenate/1
  Selector5/1 -> Vector Concatenate1/3
  Selector7/1 -> Vector Concatenate2/2
  Vector Concatenate2/1 -> Out3/1
  Vector Concatenate1/1 -> Out2/1
  Selector1/1 -> Vector Concatenate/2
  Selector3/1 -> Vector Concatenate1/1

== system massbalancer3/TNet/Subsystem1/Term3/X ==
  ddoubledot : Inport
  s : Inport  Port=2
  r : Inport  Port=3
  Cross Product : matrix_library/Cross Product
  Display : Display
  Display1 : Display
  Display2 : Display
  Product : Product
  y : Outport
  wires:
  Cross Product/1 -> y/1
  ddoubledot/1 -> Display2/1, Product/1
  Product/1 -> Display/1, Cross Product/2
  r/1 -> Cross Product/1
  s/1 -> Product/2, Display1/1

== system massbalancer3/TNet/Subsystem1/Term3/Y ==
  ddoubledot : Inport
  s : Inport  Port=2
  r : Inport  Port=3
  Cross Product : matrix_library/Cross Product
  Display : Display
  Product : Product
  y : Outport
  wires:
  Cross Product/1 -> y/1
  ddoubledot/1 -> Product/1
  Product/1 -> Cross Product/2
  r/1 -> Display/1, Cross Product/1
  s/1 -> Product/2

== system massbalancer3/TNet/Subsystem1/Term3/Z ==
  r : Inport
  s : Inport  Port=2
  ddoubledot : Inport  Port=3
  Cross Product : matrix_library/Cross Product
  Display : Display
  Display1 : Display
  Product : Product
  y : Outport
  wires:
  Cross Product/1 -> Display/1, y/1
  ddoubledot/1 -> Display1/1, Product/1
  s/1 -> Product/2
  Product/1 -> Cross Product/2
  r/1 -> Cross Product/1

== system massbalancer3/TNet/TBalances/R_I/Subsystem3 ==
  In1 : Inport
  Reshape : Reshape  OutputDimensionality=Column vector (2-D)  OutputDimensions=[1,3]
  Selector : Selector  InputPortWidth=9  IndexOptions=Index vector (dialog)  Indices=[1]  OutputSizes=1
  Selector1 : Selector  InputPortWidth=9  IndexOptions=Index vector (dialog)  Indices=[2]  OutputSizes=1
  Selector2 : Selector  InputPortWidth=9  IndexOptions=Index vector (dialog)  Indices=[3]  OutputSizes=1
  Selector3 : Selector  InputPortWidth=9  IndexOptions=Index vector (dialog)  Indices=[4]  OutputSizes=1
  Selector4 : Selector  InputPortWidth=9  IndexOptions=Index vector (dialog)  Indices=[5]  OutputSizes=1
  Selector5 : Selector  InputPortWidth=9  IndexOptions=Index vector (dialog)  Indices=[6]  OutputSizes=1
  Selector6 : Selector  InputPortWidth=9  IndexOptions=Index vector (dialog)  Indices=[7]  OutputSizes=1
  Selector7 : Selector  InputPortWidth=9  IndexOptions=Index vector (dialog)  Indices=[8]  OutputSizes=1
  Selector8 : Selector  InputPortWidth=9  IndexOptions=Index vector (dialog)  Indices=[9]  OutputSizes=1
  Vector Concatenate : Concatenate  NumInputs=3  Mode=Multidimensional array
  Vector Concatenate1 : Concatenate  NumInputs=3  Mode=Multidimensional array
  Vector Concatenate2 : Concatenate  NumInputs=3  Mode=Multidimensional array
  Out1 : Outport
  Out2 : Outport  Port=2
  Out3 : Outport  Port=3
  wires:
  Selector2/1 -> Vector Concatenate/3
  Vector Concatenate/1 -> Out1/1
  Selector8/1 -> Vector Concatenate2/3
  Selector4/1 -> Vector Concatenate1/2
  Selector6/1 -> Vector Concatenate2/1
  In1/1 -> Reshape/1
  Reshape/1 -> Selector8/1, Selector7/1, Selector6/1, Selector5/1, Selector4/1, Selector3/1, Selector2/1, Selector1/1, Selector/1
  Selector/1 -> Vector Concatenate/1
  Selector5/1 -> Vector Concatenate1/3
  Selector7/1 -> Vector Concatenate2/2
  Vector Concatenate2/1 -> Out3/1
  Vector Concatenate1/1 -> Out2/1
  Selector1/1 -> Vector Concatenate/2
  Selector3/1 -> Vector Concatenate1/1

== system massbalancer3/TNet/TBalances/R_I/Subsystem4 ==
  In1 : Inport
  Reshape : Reshape  OutputDimensionality=Column vector (2-D)  OutputDimensions=[1,3]
  Selector : Selector  InputPortWidth=9  IndexOptions=Index vector (dialog)  Indices=[1]  OutputSizes=1
  Selector1 : Selector  InputPortWidth=9  IndexOptions=Index vector (dialog)  Indices=[2]  OutputSizes=1
  Selector2 : Selector  InputPortWidth=9  IndexOptions=Index vector (dialog)  Indices=[3]  OutputSizes=1
  Selector3 : Selector  InputPortWidth=9  IndexOptions=Index vector (dialog)  Indices=[4]  OutputSizes=1
  Selector4 : Selector  InputPortWidth=9  IndexOptions=Index vector (dialog)  Indices=[5]  OutputSizes=1
  Selector5 : Selector  InputPortWidth=9  IndexOptions=Index vector (dialog)  Indices=[6]  OutputSizes=1
  Selector6 : Selector  InputPortWidth=9  IndexOptions=Index vector (dialog)  Indices=[7]  OutputSizes=1
  Selector7 : Selector  InputPortWidth=9  IndexOptions=Index vector (dialog)  Indices=[8]  OutputSizes=1
  Selector8 : Selector  InputPortWidth=9  IndexOptions=Index vector (dialog)  Indices=[9]  OutputSizes=1
  Vector Concatenate : Concatenate  NumInputs=3  Mode=Multidimensional array
  Vector Concatenate1 : Concatenate  NumInputs=3  Mode=Multidimensional array
  Vector Concatenate2 : Concatenate  NumInputs=3  Mode=Multidimensional array
  Out1 : Outport
  Out2 : Outport  Port=2
  Out3 : Outport  Port=3
  wires:
  Selector3/1 -> Vector Concatenate1/1
  Selector1/1 -> Vector Concatenate/2
  Vector Concatenate1/1 -> Out2/1
  Vector Concatenate2/1 -> Out3/1
  Selector7/1 -> Vector Concatenate2/2
  Selector5/1 -> Vector Concatenate1/3
  Selector/1 -> Vector Concatenate/1
  Reshape/1 -> Selector/1, Selector1/1, Selector2/1, Selector3/1, Selector4/1, Selector5/1, Selector6/1, Selector7/1, Selector8/1
  In1/1 -> Reshape/1
  Selector6/1 -> Vector Concatenate2/1
  Selector4/1 -> Vector Concatenate1/2
  Selector8/1 -> Vector Concatenate2/3
  Vector Concatenate/1 -> Out1/1
  Selector2/1 -> Vector Concatenate/3

== system massbalancer3/TNet/TBalances/Term1/Subsystem1 ==
  R_0 : Inport
  Reshape : Reshape  OutputDimensionality=Column vector (2-D)  OutputDimensions=[1,3]
  Selector : Selector  InputPortWidth=9  IndexOptions=Index vector (dialog)  Indices=[1]  OutputSizes=1
  Selector1 : Selector  InputPortWidth=9  IndexOptions=Index vector (dialog)  Indices=[2]  OutputSizes=1
  Selector2 : Selector  InputPortWidth=9  IndexOptions=Index vector (dialog)  Indices=[3]  OutputSizes=1
  Selector3 : Selector  InputPortWidth=9  IndexOptions=Index vector (dialog)  Indices=[4]  OutputSizes=1
  Selector4 : Selector  InputPortWidth=9  IndexOptions=Index vector (dialog)  Indices=[5]  OutputSizes=1
  Selector5 : Selector  InputPortWidth=9  IndexOptions=Index vector (dialog)  Indices=[6]  OutputSizes=1
  Selector6 : Selector  InputPortWidth=9  IndexOptions=Index vector (dialog)  Indices=[7]  OutputSizes=1
  Selector7 : Selector  InputPortWidth=9  IndexOptions=Index vector (dialog)  Indices=[8]  OutputSizes=1
  Selector8 : Selector  InputPortWidth=9  IndexOptions=Index vector (dialog)  Indices=[9]  OutputSizes=1
  Vector Concatenate : Concatenate  NumInputs=3  Mode=Multidimensional array
  Vector Concatenate1 : Concatenate  NumInputs=3  Mode=Multidimensional array
  Vector Concatenate2 : Concatenate  NumInputs=3  Mode=Multidimensional array
  Out1 : Outport
  Out2 : Outport  Port=2
  Out3 : Outport  Port=3
  wires:
  Selector3/1 -> Vector Concatenate1/1
  Selector1/1 -> Vector Concatenate/2
  Vector Concatenate1/1 -> Out2/1
  Vector Concatenate2/1 -> Out3/1
  Selector7/1 -> Vector Concatenate2/2
  Selector5/1 -> Vector Concatenate1/3
  Selector/1 -> Vector Concatenate/1
  Reshape/1 -> Selector/1, Selector1/1, Selector2/1, Selector3/1, Selector4/1, Selector5/1, Selector6/1, Selector7/1, Selector8/1
  R_0/1 -> Reshape/1
  Selector6/1 -> Vector Concatenate2/1
  Selector4/1 -> Vector Concatenate1/2
  Selector8/1 -> Vector Concatenate2/3
  Vector Concatenate/1 -> Out1/1
  Selector2/1 -> Vector Concatenate/3

== system massbalancer3/TNet/TBalances/Term1/Subsystem3 ==
  R_0 : Inport
  Reshape : Reshape  OutputDimensionality=Column vector (2-D)  OutputDimensions=[1,3]
  Selector : Selector  InputPortWidth=9  IndexOptions=Index vector (dialog)  Indices=[1]  OutputSizes=1
  Selector1 : Selector  InputPortWidth=9  IndexOptions=Index vector (dialog)  Indices=[2]  OutputSizes=1
  Selector2 : Selector  InputPortWidth=9  IndexOptions=Index vector (dialog)  Indices=[3]  OutputSizes=1
  Selector3 : Selector  InputPortWidth=9  IndexOptions=Index vector (dialog)  Indices=[4]  OutputSizes=1
  Selector4 : Selector  InputPortWidth=9  IndexOptions=Index vector (dialog)  Indices=[5]  OutputSizes=1
  Selector5 : Selector  InputPortWidth=9  IndexOptions=Index vector (dialog)  Indices=[6]  OutputSizes=1
  Selector6 : Selector  InputPortWidth=9  IndexOptions=Index vector (dialog)  Indices=[7]  OutputSizes=1
  Selector7 : Selector  InputPortWidth=9  IndexOptions=Index vector (dialog)  Indices=[8]  OutputSizes=1
  Selector8 : Selector  InputPortWidth=9  IndexOptions=Index vector (dialog)  Indices=[9]  OutputSizes=1
  Vector Concatenate : Concatenate  NumInputs=3  Mode=Multidimensional array
  Vector Concatenate1 : Concatenate  NumInputs=3  Mode=Multidimensional array
  Vector Concatenate2 : Concatenate  NumInputs=3  Mode=Multidimensional array
  Out1 : Outport
  Out2 : Outport  Port=2
  Out3 : Outport  Port=3
  wires:
  Selector2/1 -> Vector Concatenate/3
  Vector Concatenate/1 -> Out1/1
  Selector8/1 -> Vector Concatenate2/3
  Selector4/1 -> Vector Concatenate1/2
  Selector6/1 -> Vector Concatenate2/1
  R_0/1 -> Reshape/1
  Reshape/1 -> Selector8/1, Selector7/1, Selector6/1, Selector5/1, Selector4/1, Selector3/1, Selector2/1, Selector1/1, Selector/1
  Selector/1 -> Vector Concatenate/1
  Selector5/1 -> Vector Concatenate1/3
  Selector7/1 -> Vector Concatenate2/2
  Vector Concatenate2/1 -> Out3/1
  Vector Concatenate1/1 -> Out2/1
  Selector1/1 -> Vector Concatenate/2
  Selector3/1 -> Vector Concatenate1/1

== system massbalancer3/TNet/TBalances/Term1/X ==
  R-0 : Inport
  dd : Inport  Port=2
  s : Inport  Port=3
  Wb : Inport  Port=4
  Cross Product : matrix_library/Cross Product
  Cross Product1 : matrix_library/Cross Product
  Display : Display
  Product : Product
  y : Outport
  wires:
  Product/1 -> Cross Product1/1
  Cross Product/1 -> Cross Product1/2
  Wb/1 -> Cross Product/1
  R-0/1 -> Cross Product/2
  Cross Product1/1 -> Display/1, y/1
  s/1 -> Product/2
  dd/1 -> Product/1

== system massbalancer3/TNet/TBalances/Term1/Y ==
  R0 : Inport
  ddot : Inport  Port=2
  s : Inport  Port=3
  Wb : Inport  Port=4
  Cross Product : matrix_library/Cross Product
  Cross Product1 : matrix_library/Cross Product
  Display : Display
  Product : Product
  y : Outport
  wires:
  R0/1 -> Cross Product/2
  Wb/1 -> Cross Product/1
  s/1 -> Product/1
  Cross Product/1 -> Cross Product1/2
  Product/1 -> Cross Product1/1
  Cross Product1/1 -> Display/1, y/1
  ddot/1 -> Product/2

== system massbalancer3/TNet/TBalances/Term1/Z ==
  ddot : Inport
  R0 : Inport  Port=2
  s : Inport  Port=3
  Wb : Inport  Port=4
  Cross Product : matrix_library/Cross Product
  Cross Product1 : matrix_library/Cross Product
  Product : Product
  y : Outport
  wires:
  ddot/1 -> Product/2
  Cross Product1/1 -> y/1
  Product/1 -> Cross Product1/1
  Cross Product/1 -> Cross Product1/2
  s/1 -> Product/1
  Wb/1 -> Cross Product/1
  R0/1 -> Cross Product/2
